simulink model "motor_"  (Simulink 6.1)
settings: Solver=ode45  StartTime=0.0  StopTime=100  RelTol=1e-3
values from neighbouring files (symbols this model uses):
  ambient = am    [Elec_Engg_10_03_01.m]    (also in Elec_Engg_10_03_011.m)
  temp_rpm = [15 16 17 18 19 20 21 22 23 24 25 26 ... (42 elements, 21x2)]    [var.mat]
libraries: simulink x1
settings Model: LastModifiedBy=vijay
settings DebuggingCC: SolverPrmCheckMsg=warning

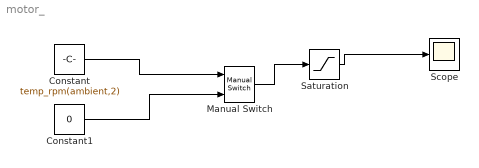
== system motor_ ==
  Constant : Constant  Value=temp_rpm(ambient,2)
  Constant1 : Constant  Value=0
  Manual Switch : simulink/Signal Routing/Manual Switch  sw=1  action=0
  Saturation : Saturate  UpperLimit=temp_rpm(ambient-14,2)  LowerLimit=-temp_rpm(ambient-14,2)
  Scope : Scope
  wires:
  Saturation/1 -> Scope/1
  Constant/1 -> Manual Switch/1
  Constant1/1 -> Manual Switch/2
  Manual Switch/1 -> Saturation/1
